simulink model "PhaseSequenceCorrector"  (R2024a)
settings: Solver=VariableStepAuto  StartTime=0.0  StopTime=1  RelTol=1e-3
libraries: sps_lib x1
settings Model: Creator=dogba  LastModifiedBy=dogba

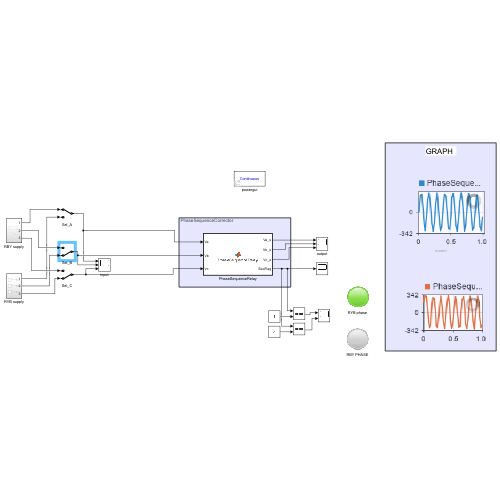
[thumbnail: Simulink's stored preview of the top-level diagram]
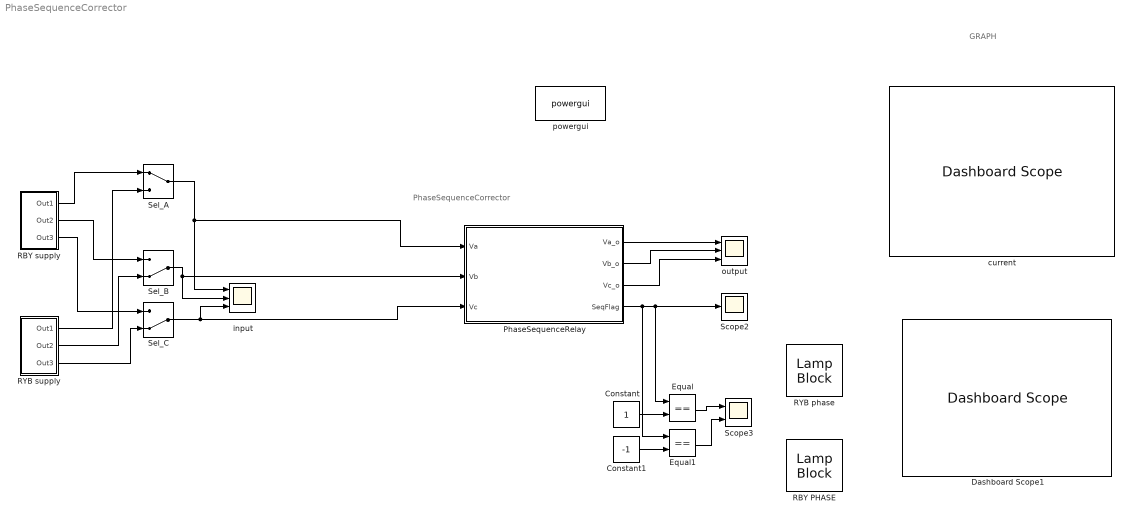
== system PhaseSequenceCorrector ==
  note: PhaseSequenceCorrector
  note: GRAPH
  Constant : Constant
  Constant1 : Constant  Value=-1
  Dashboard Scope1 : DashboardScope
  Equal : RelationalOperator  Operator===  OutDataTypeStr=boolean  RndMeth=Simplest  InputSameDT=off
  Equal1 : RelationalOperator  Operator===  OutDataTypeStr=boolean  RndMeth=Simplest  InputSameDT=off
  PhaseSequenceRelay : MATLAB Function  TreatAsAtomicUnit=on
  RBY PHASE : LampBlock  LabelPosition=Hide
  RBY supply : Subsystem
  RYB phase : LampBlock  LabelPosition=Hide
  RYB supply : Subsystem
  Scope2 : Scope
  Scope3 : Scope  NumInputPorts=2
  Sel_A : ManualSwitch
  Sel_B : ManualSwitch  CurrentSetting=0
  Sel_C : ManualSwitch  CurrentSetting=0
  current : DashboardScope
  input : Scope  NumInputPorts=3
  output : Scope  NumInputPorts=3
  powergui : sps_lib/powergui  Priority=1  SimulationMode=Continuous  SampleTime=50e-6  frequency=60  Iterations=50  frequencyindice=60  Pbase=100e6  ErrMax=1e-4  UnitsV=kV  UnitsW=MW  buscounter=0  FunctionMessages=off  echomessages=off  EnableUseOfTLC=off  CurrentSourceSwitches=off  DisableSnubberDevices=off  DisableRonSwitches=off  DisableVfSwitches=off  DisplayEquations=off  AutomaticDiscreteSolvers=off  SolverType=Tustin/Backward Euler (TBE)  Interpol=off  ExternalGateDelay=off  methode=off  Ts=100  x0status=blocks  SPID=on  SwTol=0  HookPort=off  NonlinearTolerance=1e-4  nMaxIteration=100  ContinueOnMaxIteration=off  RestoreLinks=warning  ResistiveCurrentMeasurement=off  Frange=[0:2:500]  Ylog=off  Xlog=on  ShowGrid=off  save=off  variable=ZData  structure=0  ZoomFFT=off  StartTime=0.0  cycles=1  DisplayStyle=1  fundamental=60  FreqAxis=off  MaxFrequency=1000  frequencyindicesteady=1  RmsSteady=1  display=off
  wires:
  PhaseSequenceRelay/1(Va_o) -> output/1
  PhaseSequenceRelay/2(Vb_o) -> output/2
  PhaseSequenceRelay/3(Vc_o) -> output/3
  RYB supply/1(Out1) -> Sel_A/2
  RYB supply/2(Out2) -> Sel_B/2
  RYB supply/3(Out3) -> Sel_C/2
  RBY supply/1(Out1) -> Sel_A/1
  RBY supply/2(Out2) -> Sel_B/1
  RBY supply/3(Out3) -> Sel_C/1
  Sel_A/1 -> PhaseSequenceRelay/1(Va), input/1
  Sel_B/1 -> PhaseSequenceRelay/2(Vb), input/2
  Sel_C/1 -> PhaseSequenceRelay/3(Vc), input/3
  Constant/1 -> Equal/2
  Equal/1 -> Scope3/1
  PhaseSequenceRelay/4(SeqFlag) -> Equal1/1, Equal/1, Scope2/1
  Constant1/1 -> Equal1/2
  Equal1/1 -> Scope3/2

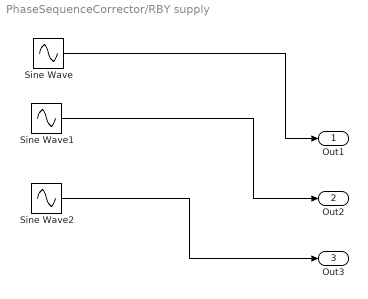
== system PhaseSequenceCorrector/RBY supply ==
  Sine Wave : Sin  Amplitude=311.111  Frequency=50  SampleTime=0
  Sine Wave1 : Sin  Amplitude=311.11  Frequency=50  Phase=120  SampleTime=0
  Sine Wave2 : Sin  Amplitude=311.111  Frequency=50  Phase=-120  SampleTime=0
  Out1 : Outport
  Out2 : Outport  Port=2
  Out3 : Outport  Port=3
  wires:
  Sine Wave2/1 -> Out3/1
  Sine Wave/1 -> Out1/1
  Sine Wave1/1 -> Out2/1

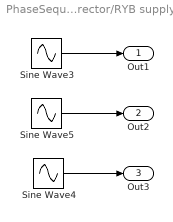
== system PhaseSequenceCorrector/RYB supply ==
  Sine Wave3 : Sin  Amplitude=311.111  Frequency=50  SampleTime=0
  Sine Wave4 : Sin  Amplitude=311.11  Frequency=50  Phase=120  SampleTime=0
  Sine Wave5 : Sin  Amplitude=311.111  Frequency=50  Phase=-120  SampleTime=0
  Out1 : Outport
  Out2 : Outport  Port=2
  Out3 : Outport  Port=3
  wires:
  Sine Wave5/1 -> Out2/1
  Sine Wave4/1 -> Out3/1
  Sine Wave3/1 -> Out1/1

== matlab function PhaseSequenceCorrector/PhaseSequenceRelay ==
  data: Va input; Va_o output; Vb input; Vc input; Vb_o output; Vc_o output; SeqFlag output
function [Va_o, Vb_o, Vc_o, SeqFlag] = PhaseSequenceRelay(Va, Vb, Vc)
%#codegen
% Detects 3-phase sequence (ABC or ACB) and corrects to ABC.
% 
% Inputs:
%   Va, Vb, Vc  - Instantaneous phase voltages (or currents)
% Outputs:
%   Va_o, Vb_o, Vc_o - Corrected 3-phase signals (always ABC order)
%   SeqFlag          - +1 for ABC, -1 for ACB

persistent theta_prev dtheta_filt init
if isempty(init)
    theta_prev = 0;
    dtheta_filt = 0;
    init = true;
end

%% Clarke Transform (αβ frame)
alpha = (2/3) * (Va - 0.5*Vb - 0.5*Vc);
beta  = (2/3) * (0.8660254037844386) * (Vb - Vc); % sqrt(3)/2

%% Electrical angle of the space vector
theta = atan2(beta, alpha);

%% Angle change per sample (wrapped to [-pi, pi])
dtheta = theta - theta_prev;
if dtheta >  pi
    dtheta = dtheta - 2*pi;
elseif dtheta < -pi
    dtheta = dtheta + 2*pi;
end
theta_prev = theta;

%% Low-pass filter the angular velocity (for stability)
alpha_f = 0.05; % smoothing factor (0 < alpha_f <= 1)
dtheta_filt = (1 - alpha_f)*dtheta_filt + alpha_f*dtheta;

%% Detect sequence & correct if needed
if dtheta_filt >= 0
    % Normal ABC sequence
    SeqFlag = int8(1);
    Va_o = Va;
    Vb_o = Vb;
    Vc_o = Vc;
else
    % Reverse ACB sequence → swap B and C
    SeqFlag = int8(-1);
    Va_o = Va;
    Vb_o = Vc;
    Vc_o = Vb;
end
